simulink model "modelo_SAS_facil_sencillo_elegante"  (R2022b)
settings: Solver=VariableStepAuto  StartTime=0.0  StopTime=340  RelTol=1e-3
values from neighbouring files (symbols this model uses):
  FT_lat = FT_lat_function_elegante(p)    [SAS.m]
settings Model: Creator=raulm  LastModifiedBy=abelu
settings ModelReferenceCC: EnableRefExpFcnMdlSchedulingChecks=on

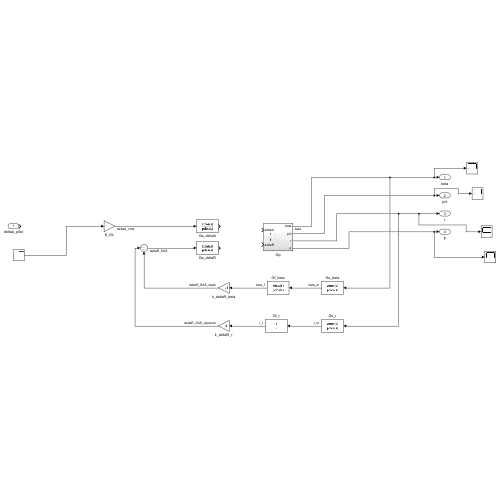
[thumbnail: Simulink's stored preview of the top-level diagram]
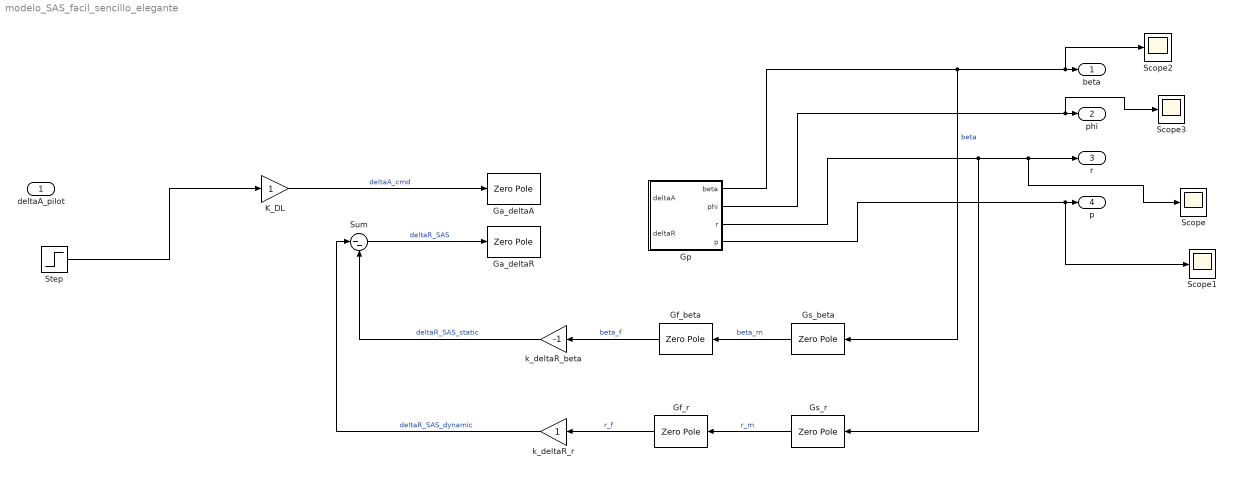
== system modelo_SAS_facil_sencillo_elegante ==
  deltaA_pilot : Inport
  Ga_deltaA : ZeroPole  Poles=[1]
  Ga_deltaR : ZeroPole  Poles=[1]
  Gf_beta : ZeroPole  Zeros=[0]  Poles=[0]
  Gf_r : ZeroPole  Zeros=[0]  Poles=0  Gain=1
  Gp : Subsystem
  Gs_beta : ZeroPole  Poles=[1]
  Gs_r : ZeroPole  Poles=[1]
  K_DL : Gain
  Scope{,1..3} (4 alike) : Scope
  Step : Step  SampleTime=0
  Sum : Sum  Inputs=|--
  k_deltaR_beta : Gain  Gain=-1
  k_deltaR_r : Gain
  beta : Outport
  phi : Outport  Port=2
  r : Outport  Port=3
  p : Outport  Port=4
  wires:
  Gp/3(r) -> Scope/1, r/1, Gs_r/1
  k_deltaR_r/1 -> Sum/1  "deltaR_SAS_dynamic"
  K_DL/1 -> Ga_deltaA/1  "deltaA_cmd"
  Gs_beta/1 -> Gf_beta/1  "beta_m"
  Gf_r/1 -> k_deltaR_r/1  "r_f"
  Gs_r/1 -> Gf_r/1  "r_m"
  Gf_beta/1 -> k_deltaR_beta/1  "beta_f"
  Gp/2(phi) -> Scope3/1, phi/1
  Gp/1(beta) -> Scope2/1, beta/1, Gs_beta/1  "beta"
  Gp/4(p) -> Scope1/1, p/1
  k_deltaR_beta/1 -> Sum/2  "deltaR_SAS_static"
  Step/1 -> K_DL/1
  Sum/1 -> Ga_deltaR/1  "deltaR_SAS"

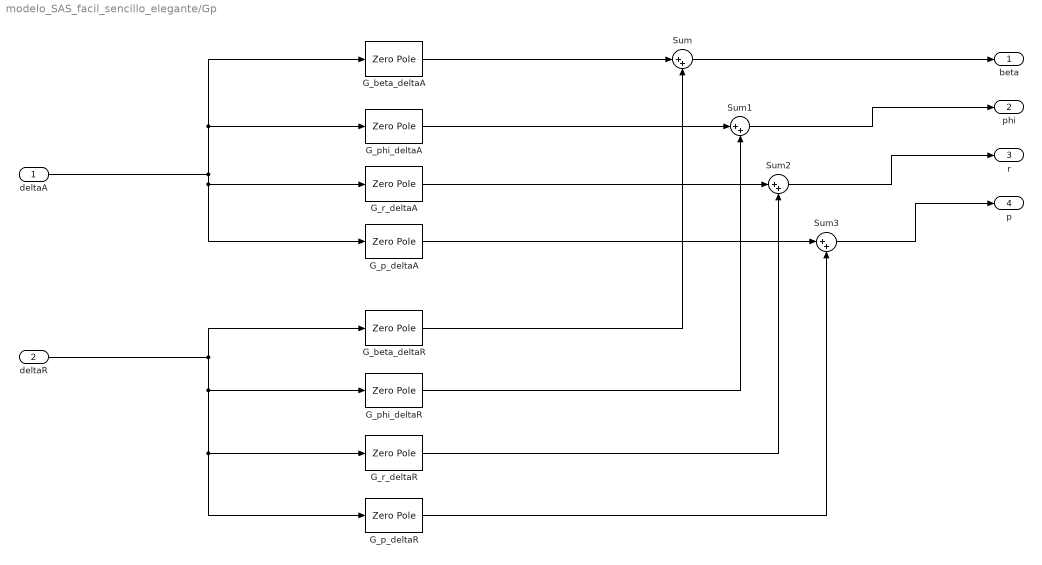
== system modelo_SAS_facil_sencillo_elegante/Gp ==
  deltaA : Inport
  deltaR : Inport  Port=2
  G_beta_deltaA : ZeroPole  Zeros=FT_lat.fact.deltaA_beta.Z{1}  Poles=FT_lat.fact.deltaA_beta.P{1}  Gain=FT_lat.fact.deltaA_beta.K
  G_beta_deltaR : ZeroPole  Zeros=FT_lat.fact.deltaR_beta.Z{1}  Poles=FT_lat.fact.deltaR_beta.P{1}  Gain=FT_lat.fact.deltaR_beta.K
  G_p_deltaA : ZeroPole  Zeros=FT_lat.fact.deltaA_p.Z{1}  Poles=FT_lat.fact.deltaA_p.P{1}  Gain=FT_lat.fact.deltaA_p.K
  G_p_deltaR : ZeroPole  Zeros=FT_lat.fact.deltaR_p.Z{1}  Poles=FT_lat.fact.deltaR_p.P{1}  Gain=FT_lat.fact.deltaR_p.K
  G_phi_deltaA : ZeroPole  Zeros=FT_lat.fact.deltaA_phi.Z{1}  Poles=FT_lat.fact.deltaA_phi.P{1}  Gain=FT_lat.fact.deltaA_phi.K
  G_phi_deltaR : ZeroPole  Zeros=FT_lat.fact.deltaR_phi.Z{1}  Poles=FT_lat.fact.deltaR_phi.P{1}  Gain=FT_lat.fact.deltaR_phi.K
  G_r_deltaA : ZeroPole  Zeros=FT_lat.fact.deltaA_r.Z{1}  Poles=FT_lat.fact.deltaA_r.P{1}  Gain=FT_lat.fact.deltaA_r.K
  G_r_deltaR : ZeroPole  Zeros=FT_lat.fact.deltaR_r.Z{1}  Poles=FT_lat.fact.deltaR_r.P{1}  Gain=FT_lat.fact.deltaR_r.K
  Sum{,1..3} (4 alike) : Sum  Inputs=|++
  beta : Outport
  phi : Outport  Port=2
  r : Outport  Port=3
  p : Outport  Port=4
  wires:
  deltaR/1 -> G_p_deltaR/1, G_r_deltaR/1, G_phi_deltaR/1, G_beta_deltaR/1
  G_phi_deltaA/1 -> Sum1/1
  deltaA/1 -> G_p_deltaA/1, G_r_deltaA/1, G_phi_deltaA/1, G_beta_deltaA/1
  G_r_deltaR/1 -> Sum2/2
  G_p_deltaA/1 -> Sum3/1
  G_r_deltaA/1 -> Sum2/1
  G_beta_deltaR/1 -> Sum/2
  Sum2/1 -> r/1
  Sum3/1 -> p/1
  Sum/1 -> beta/1
  G_p_deltaR/1 -> Sum3/2
  Sum1/1 -> phi/1
  G_beta_deltaA/1 -> Sum/1
  G_phi_deltaR/1 -> Sum1/2
